simulink model "Model_6DOF_B3"  (R2020b)
settings: Solver=FixedStepAuto  StartTime=0.0  StopTime=120  FixedStep=0.05  RelTol=1e-3
values from neighbouring files (symbols this model uses):
  Ba_0 = [0 0 0 0 0 0]    [ctrl_mode_param.m]
  Bb = 4418825.3321    [load_data.m]
  Bv_0 = [tgt_speed 0 0 0 0 0]    [ctrl_mode_param.m]
  Bx_0 = [0 0 tgt_depth 0 0 0]    [ctrl_mode_param.m]
  Ixx = 5.23e7    (= 52300000)    [load_data.m]
  Ixy = 0    [load_data.m]
  Ixz = 0    [load_data.m]
  Iyy = 1.375e9    (= 1375000000)    [load_data.m]
  Iyz = 0    [load_data.m]
  Izz = 1.367e9    (= 1367000000)    [load_data.m]
  Mb = 4418825.3321    [load_data.m]
  Xb = 0    [load_data.m]
  Xg = 0    [load_data.m]
  Yb = 0    [load_data.m]
  Yg = 0    [load_data.m]
  Zb = 0.4406    [load_data.m]
  Zg = 0    [load_data.m]
undefined symbols (not defined in the file or in its folder): dA_BP1, dA_BP2, dA_Hull, dA_PH, dA_Sail, dA_SProot, dA_X1a, dA_X1b, dA_X2a, dA_X2b, dA_X3a, dA_X3b, dA_X4a, dA_X4b, its, n_BP1, n_BP2, n_Hull, n_PH, n_Sail, n_SProot, n_X1a, n_X1b, n_X2a, n_X2b, n_X3a, n_X3b, n_X4a, n_X4b, nt_BP1, nt_BP2, nt_Hull, nt_PH, nt_Sail, nt_SProot, nt_X1a, nt_X1b, nt_X2a, nt_X2b, nt_X3a, nt_X3b, nt_X4a, nt_X4b, Usp, vt1_BP1, vt1_BP2, vt1_Hull, vt1_PH, vt1_Sail, vt1_SProot, vt1_X1a, vt1_X1b, vt1_X2a, vt1_X2b, vt1_X3a, vt1_X3b, vt1_X4a, vt1_X4b, vt2_BP1, vt2_BP2 ... (+27)
libraries: simulink x5
(part 1 of 15)
settings Model: OrderedModelArguments=off  Creator=yagkim  LastModifiedBy=cooki
settings DebuggingCC: UnderSpecifiedDimensionMsg=warning
settings SFSimCC: CustomCodeUndefinedFunction=UseInterfaceOnly

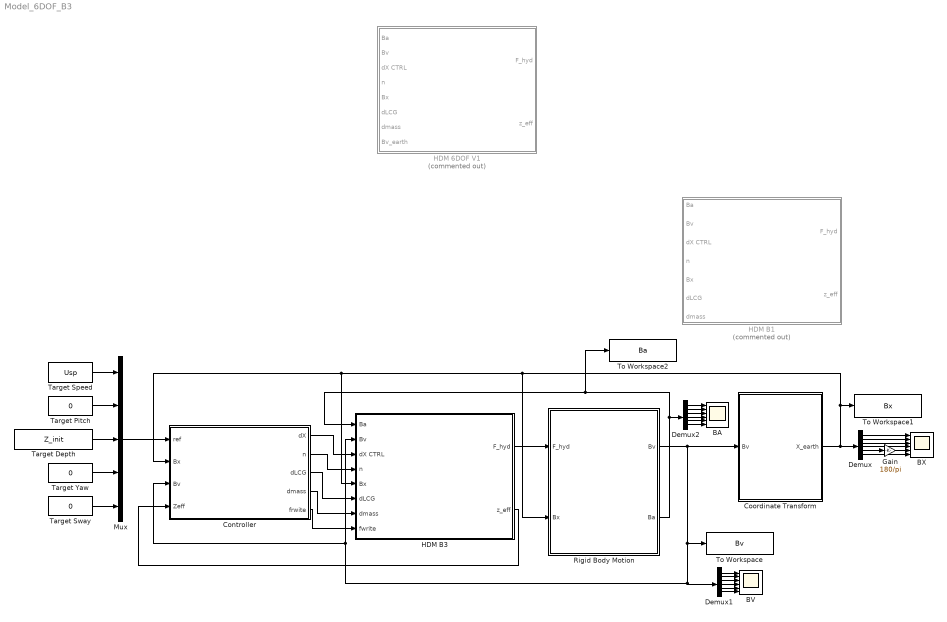
== system Model_6DOF_B3 ==
  BA : Scope  NumInputPorts=6
  BV : Scope  NumInputPorts=6
  BX : Scope  NumInputPorts=6
  Controller : Subsystem
  Coordinate Transform : Subsystem
  Demux : Demux  Outputs=6
  Demux1 : Demux  Outputs=6
  Demux2 : Demux  Outputs=6
  Gain : Gain  Gain=180/pi
  HDM 6DOF V1 : Subsystem  Commented=on  InitFcn='main'
  HDM B1 : Subsystem  Commented=on  InitFcn='main'
  HDM B3 : Subsystem  InitFcn='main'
  Mux : Mux  Inputs=5
  Rigid Body Motion : Subsystem
  Target Depth : Constant  Value=Z_init
  Target Pitch : Constant  Value=0
  Target Speed : Constant  Value=Usp
  Target Sway : Constant  Value=0
  Target Yaw : Constant  Value=0
  To Workspace : ToWorkspace  VariableName=Bv  SaveFormat=Timeseries  SampleTime=-1
  To Workspace1 : ToWorkspace  VariableName=Bx  SaveFormat=Timeseries  SampleTime=-1
  To Workspace2 : ToWorkspace  VariableName=Ba  SaveFormat=Timeseries  SampleTime=-1
  wires:
  Demux/1 -> BX/1
  Demux/2 -> BX/2
  Demux/3 -> BX/3
  Demux/4 -> BX/4
  Demux/6 -> BX/6
  Demux1/6 -> BV/6
  Demux1/5 -> BV/5
  Demux1/4 -> BV/4
  Demux1/3 -> BV/3
  Demux1/2 -> BV/2
  Demux1/1 -> BV/1
  Mux/1 -> Controller/1(ref)
  Target Speed/1 -> Mux/1
  Target Depth/1 -> Mux/3
  Gain/1 -> BX/5
  Demux/5 -> Gain/1
  Controller/2(n) -> HDM B3/4(n)
  Demux2/4 -> BA/4
  Demux2/1 -> BA/1
  Demux2/3 -> BA/3
  Demux2/6 -> BA/6
  Demux2/5 -> BA/5
  Demux2/2 -> BA/2
  Rigid Body Motion/2(Ba) -> To Workspace2/1, HDM B3/1(Ba), Demux2/1
  Rigid Body Motion/1(Bv) -> Coordinate Transform/1(Bv), Demux1/1, HDM B3/2(Bv), Controller/3(Bv), To Workspace/1
  HDM B3/1(F_hyd) -> Rigid Body Motion/1(F_hyd)
  Target Pitch/1 -> Mux/2
  Target Yaw/1 -> Mux/4
  Target Sway/1 -> Mux/5
  Coordinate Transform/1(X_earth) -> Demux/1, Rigid Body Motion/2(Bx), Controller/2(Bx), HDM B3/5(Bx), To Workspace1/1
  Controller/1(dX) -> HDM B3/3(dX CTRL)
  Controller/3(dLCG) -> HDM B3/6(dLCG)
  Controller/4(dmass) -> HDM B3/7(dmass)
  HDM B3/2(z_eff) -> Controller/4(Zeff)
  Controller/5(frwite) -> HDM B3/8(fwrite)

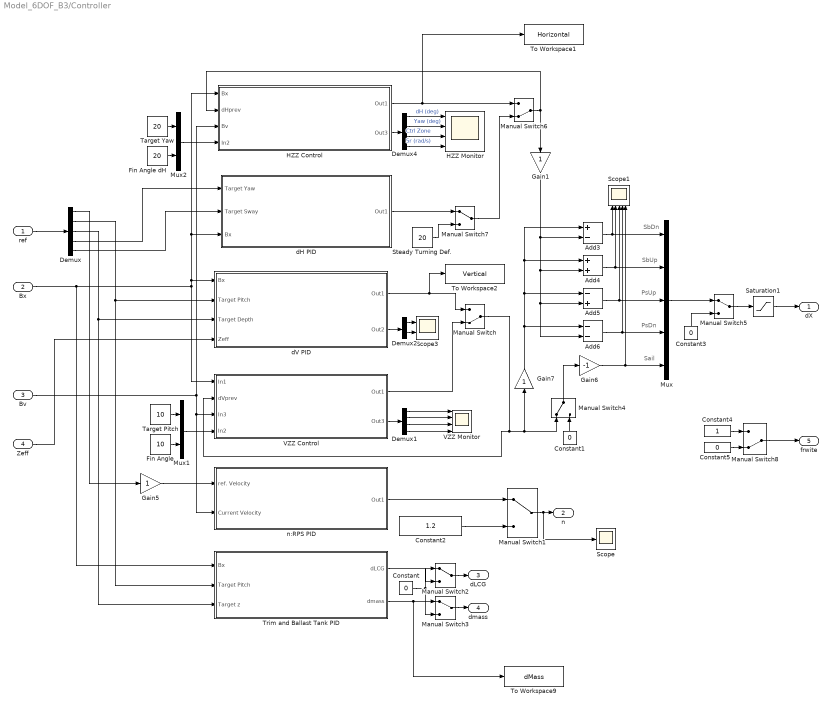
== system Model_6DOF_B3/Controller ==
  note: SbDn
  note: SbUp
  note: PsUp
  note: PsDn
  note: Sail
  ref : Inport
  Bx : Inport  Port=2
  Bv : Inport  Port=3
  Zeff : Inport  Port=4
  Add3 : Sum  Inputs=+-
  Add4 : Sum
  Add5 : Sum  Inputs=-+
  Add6 : Sum  Inputs=--
  Constant{,1,3,5} (4 alike) : Constant  Value=0
  Constant2 : Constant  Value=1.2
  Constant4 : Constant
  Demux : Demux  Outputs=5
  Demux1 : Demux
  Demux2 : Demux  Outputs=2
  Demux4 : Demux
  Fin Angle : Constant  Value=10
  Fin Angle dH : Constant  Value=20
  Gain1 : Gain
  Gain5 : Gain
  Gain6 : Gain  Gain=-1
  Gain7 : Gain
  HZZ Control : Subsystem
  HZZ Monitor : Scope  NumInputPorts=4
  Manual Switch : ManualSwitch  CurrentSetting=0
  Manual Switch{1..5,7} (6 alike) : ManualSwitch
  Manual Switch6 : ManualSwitch  CurrentSetting=0
  Manual Switch8 : ManualSwitch  CurrentSetting=0
  Mux : Mux  Inputs=5
  Mux1 : Mux  Inputs=2
  Mux2 : Mux  Inputs=2
  Saturation1 : Saturate  UpperLimit=30  LowerLimit=-30
  Scope : Scope
  Scope1 : Scope  NumInputPorts=5
  Scope3 : Scope  NumInputPorts=2
  Steady Turning Def. : Constant  Value=20
  Target Pitch : Constant  Value=10
  Target Yaw : Constant  Value=20
  To Workspace1 : ToWorkspace  VariableName=Horizontal  SaveFormat=Timeseries  SampleTime=-1
  To Workspace2 : ToWorkspace  VariableName=Vertical  SaveFormat=Timeseries  SampleTime=-1
  To Workspace9 : ToWorkspace  VariableName=dMass  SaveFormat=Timeseries  SampleTime=-1
  Trim and Ballast Tank PID : Subsystem
  VZZ Control : Subsystem
  VZZ Monitor : Scope  NumInputPorts=4
  dH PID : Subsystem
  dV PID : Subsystem
  n:RPS PID : Subsystem
  dX : Outport  VectorParamsAs1DForOutWhenUnconnected=off
  n : Outport  Port=2  VectorParamsAs1DForOutWhenUnconnected=off
  dLCG : Outport  Port=3  VectorParamsAs1DForOutWhenUnconnected=off
  dmass : Outport  Port=4  VectorParamsAs1DForOutWhenUnconnected=off
  frwite : Outport  Port=5  VectorParamsAs1DForOutWhenUnconnected=off
  wires:
  Add3/1 -> Mux/1, Scope1/1
  Add4/1 -> Mux/2, Scope1/2
  Add5/1 -> Mux/3, Scope1/3
  Add6/1 -> Mux/4, Scope1/4
  Manual Switch6/1 -> HZZ Control/2(dHprev), Gain1/1
  Gain6/1 -> Mux/5, Scope1/5
  Gain7/1 -> Add3/1, Add4/1, Add5/1, Add6/1
  Demux/1 -> Gain5/1
  Bv/1 -> HZZ Control/3(Bv), n:RPS PID/2(Current Velocity), VZZ Control/3(In3)
  Gain5/1 -> n:RPS PID/1(ref. Velocity)
  Constant2/1 -> Manual Switch1/2
  n:RPS PID/1(Out1) -> Manual Switch1/1
  Manual Switch/1 -> VZZ Control/2(dVprev), Manual Switch4/1, Gain7/1
  ref/1 -> Demux/1
  dV PID/1(Out1) -> Manual Switch/1, To Workspace2/1
  Demux/4 -> dH PID/1(Target Yaw)
  Demux/5 -> dH PID/2(Target Sway)
  dH PID/1(Out1) -> Manual Switch7/1
  VZZ Control/1(Out1) -> Manual Switch/2
  Demux1/1 -> VZZ Monitor/1
  Demux1/2 -> VZZ Monitor/2
  Demux1/3 -> VZZ Monitor/3
  Demux1/4 -> VZZ Monitor/4
  VZZ Control/2(Out3) -> Demux1/1
  Mux1/1 -> VZZ Control/4(In2)
  Target Pitch/1 -> Mux1/1
  Fin Angle/1 -> Mux1/2
  Demux/2 -> Trim and Ballast Tank PID/2(Target Pitch), dV PID/2(Target Pitch)
  Bx/1 -> Trim and Ballast Tank PID/1(Bx), HZZ Control/1(Bx), dH PID/3(Bx), dV PID/1(Bx), VZZ Control/1(In1)
  Demux/3 -> Trim and Ballast Tank PID/3(Target z), dV PID/3(Target Depth)
  Trim and Ballast Tank PID/1(dLCG) -> Manual Switch2/2
  Trim and Ballast Tank PID/2(dmass) -> To Workspace9/1, Manual Switch3/1
  Mux/1 -> Manual Switch5/1
  Demux2/2 -> Scope3/2
  Demux2/1 -> Scope3/1
  dV PID/2(Out2) -> Demux2/1
  Manual Switch2/1 -> dLCG/1
  Constant/1 -> Manual Switch3/2, Manual Switch2/1
  Manual Switch4/1 -> Gain6/1
  Constant1/1 -> Manual Switch4/2
  Manual Switch5/1 -> Saturation1/1
  Constant3/1 -> Manual Switch5/2
  Fin Angle dH/1 -> Mux2/2
  Mux2/1 -> HZZ Control/4(In2)
  Target Yaw/1 -> Mux2/1
  Demux4/3 -> HZZ Monitor/3  "Ctrl Zone"
  HZZ Control/2(Out3) -> Demux4/1
  Demux4/4 -> HZZ Monitor/4  "5r (rad/s)"
  Demux4/2 -> HZZ Monitor/2  "Yaw (deg)"
  Demux4/1 -> HZZ Monitor/1  "dH (deg)"
  HZZ Control/1(Out1) -> To Workspace1/1, Manual Switch6/1
  Gain1/1 -> Add6/2, Add5/2, Add4/2, Add3/2
  Zeff/1 -> dV PID/4(Zeff)
  Saturation1/1 -> dX/1
  Manual Switch1/1 -> Scope/1, n/1
  Manual Switch3/1 -> dmass/1
  Manual Switch7/1 -> Manual Switch6/2
  Steady Turning Def./1 -> Manual Switch7/2
  Manual Switch8/1 -> frwite/1
  Constant4/1 -> Manual Switch8/1
  Constant5/1 -> Manual Switch8/2

== system Model_6DOF_B3/Coordinate Transform ==
  Bv : Inport
  Demux : Demux  Outputs=6
  Gain2 : Gain
  Gain6 : Gain
  Integrator : Integrator  InitialCondition=Bx_0
  MATLAB Function2 : MATLAB Function  TreatAsAtomicUnit=on
  Mux : Mux  Inputs=6
  X_earth : Outport  VectorParamsAs1DForOutWhenUnconnected=off
  wires:
  Bv/1 -> MATLAB Function2/2(Bv)
  MATLAB Function2/1(out) -> Integrator/1
  Integrator/1 -> MATLAB Function2/1(Bx), Demux/1
  Mux/1 -> X_earth/1
  Demux/1 -> Mux/1
  Demux/2 -> Mux/2
  Demux/3 -> Gain6/1
  Demux/4 -> Mux/4
  Demux/5 -> Gain2/1
  Demux/6 -> Mux/6
  Gain6/1 -> Mux/3
  Gain2/1 -> Mux/5

== system Model_6DOF_B3/HDM 6DOF V1 ==
  Ba : Inport
  Bv : Inport  Port=2
  dX CTRL : Inport  Port=3
  n : Inport  Port=4
  Bx : Inport  Port=5
  dLCG : Inport  Port=6
  dmass : Inport  Port=7
  Bv_earth : Inport  Port=8
  Constant4 : Constant  Value=0
  Effective Veloicity Calclation : Subsystem
  Effective dX Calculation : Subsystem
  K : Subsystem
  M : Subsystem
  M 6d org : Subsystem  Commented=on
  Manual Switch1 : ManualSwitch
  Manual Switch2 : ManualSwitch
  Manual Switch3 : ManualSwitch  CurrentSetting=0
  Manual Switch4 : ManualSwitch  CurrentSetting=0
  Manual Switch5 : ManualSwitch
  Mux2 : Mux  Inputs=6
  N : Subsystem
  Sea State : Constant  Value=0
  To Workspace1 : ToWorkspace  VariableName=dXeff  SaveFormat=Timeseries  SampleTime=-1
  To Workspace2 : ToWorkspace  VariableName=AOA  SaveFormat=Timeseries  SampleTime=-1
  Wave Particle Velocity : Subsystem
  X : Subsystem
  X 6d org : Subsystem  Commented=on
  Y : Subsystem
  Z : Subsystem
  Z 6d org : Subsystem  Commented=on
  alpha : Scope
  dXeff : Scope
  F_hyd : Outport  VectorParamsAs1DForOutWhenUnconnected=off
  z_eff : Outport  Port=2  VectorParamsAs1DForOutWhenUnconnected=off
  wires:
  Constant4/1 -> Manual Switch4/2, Manual Switch3/2, Manual Switch1/1, Manual Switch2/1, Manual Switch5/1
  Mux2/1 -> F_hyd/1
  X/1(X) -> Mux2/1
  Manual Switch3/1 -> Mux2/3
  Manual Switch2/1 -> Mux2/5
  Effective dX Calculation/1(dXeff) -> To Workspace1/1, dXeff/1, X/5(dXeff), M/6(dX), K/6(dX), Z/6(dX), N/6(dX), Y/6(dX)
  Ba/1 -> X/3(Ba), Y/3(Ba), K/3(Ba), Z/3(Ba), M/3(Ba), N/3(Ba)
  M/1(M) -> Manual Switch2/2
  Z/1(Z) -> Manual Switch3/1
  dX CTRL/1 -> X/12(dXraw), Effective dX Calculation/1(dX CTRL)
  Bx/1 -> X/1(Bx), N/1(Bx), K/1(Bx), Y/1(Bx), Z/1(Bx), M/1(Bx), Wave Particle Velocity/1(Bx_earth)
  dLCG/1 -> Wave Particle Velocity/5(dLCG), X/9(dLCG), Z/8(dLCG), N/8(dLCG), M/8(dLCG), K/8(dLCG), Y/8(dLCG)
  dmass/1 -> M/9(dmass), N/9(dmass), K/9(dmass), Z/9(dmass), Y/9(dmass), X/10(dmass)
  Bv/1 -> Z/2(Bv), N/2(Bv), K/2(Bv), Y/2(Bv), Effective Veloicity Calclation/1(Bv), X/2(Bv), M/2(Bv), Wave Particle Velocity/3(Bv_ship)
  Bv_earth/1 -> Wave Particle Velocity/2(Bv_earth)
  Sea State/1 -> Wave Particle Velocity/4(SeaState)
  Wave Particle Velocity/7(z_eff) -> z_eff/1
  N/1(N) -> Manual Switch1/2
  Y/1(Y) -> Manual Switch4/1
  Manual Switch4/1 -> Mux2/2
  Manual Switch1/1 -> Mux2/6
  Manual Switch5/1 -> Mux2/4
  K/1(K) -> Manual Switch5/2
  Wave Particle Velocity/2(Yvm) -> Y/10(Yvm)
  Wave Particle Velocity/4(Kvm) -> K/10(Kvm)
  Wave Particle Velocity/6(Nvm) -> N/10(Nvm)
  Wave Particle Velocity/8(uwsXi) -> Effective Veloicity Calclation/2(uwsXi)
  Wave Particle Velocity/9(uwsCG) -> Effective Veloicity Calclation/3(uwsCG)
  Effective Veloicity Calclation/5(UeX) -> Y/7(UeX), X/6(UeSP), Z/7(UeSP), N/7(UeX), K/7(UeX), M/7(UeSP)
  Effective Veloicity Calclation/3(Umag) -> Y/5(Umag), M/5(Umag), Z/5(Umag), X/4(Umag), K/5(Umag), N/5(Umag)
  Effective Veloicity Calclation/1(Alpha) -> alpha/1, To Workspace2/1, Z/4(Alpha), M/4(Alpha), X/8(Alpha)
  Effective Veloicity Calclation/2(Beta) -> N/4(Beta), K/4(Beta), Y/4(Beta)
  Effective Veloicity Calclation/4(aXi) -> X/11(dXadd), Effective dX Calculation/2(aXi)
  Wave Particle Velocity/1(Xvm) -> X/13(Xvm)
  n/1 -> X/7(n)
  Wave Particle Velocity/3(Zvm) -> Z/10(Zvm)
  Wave Particle Velocity/5(Mvm) -> M/10(Mvm)

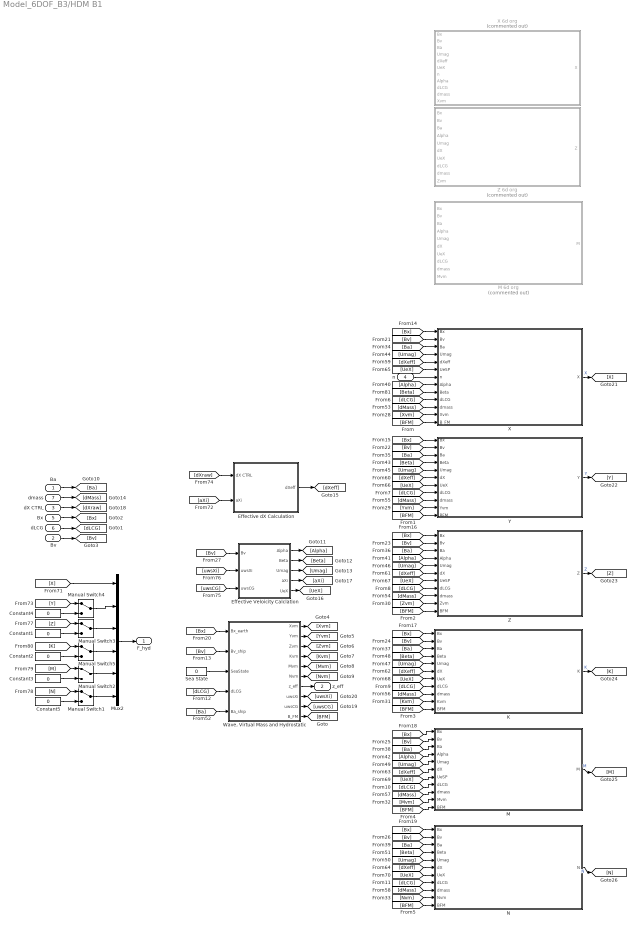
== system Model_6DOF_B3/HDM B1 ==
  Ba : Inport
  Bv : Inport  Port=2
  dX CTRL : Inport  Port=3
  n : Inport  Port=4
  Bx : Inport  Port=5
  dLCG : Inport  Port=6
  dmass : Inport  Port=7
  Constant{1..5} (5 alike) : Constant  Value=0
  Effective Veloicity Calclation : Subsystem
  Effective dX Calculation : Subsystem
  K : Subsystem
  M : Subsystem
  M 6d org : Subsystem  Commented=on
  Manual Switch{1..5} (5 alike) : ManualSwitch
  Mux2 : Mux  Inputs=6
  N : Subsystem
  Sea State : Constant  Value=0
  "Wave, Virtual Mass and Hydrostatic" : Subsystem
  X : Subsystem
  X 6d org : Subsystem  Commented=on
  Y : Subsystem
  Z : Subsystem
  Z 6d org : Subsystem  Commented=on
  F_hyd : Outport  VectorParamsAs1DForOutWhenUnconnected=off
  z_eff : Outport  Port=2  VectorParamsAs1DForOutWhenUnconnected=off
  wires:
  [Beta] -> X/9(Beta)
  [K] -> Manual Switch5/1
  [M] -> Manual Switch2/1
  [N] -> Manual Switch1/1
  [Z] -> Manual Switch3/1
  [Y] -> Manual Switch4/1
  Constant5/1 -> Manual Switch1/2
  Constant3/1 -> Manual Switch2/2
  Constant2/1 -> Manual Switch5/2
  Constant1/1 -> Manual Switch3/2
  Constant4/1 -> Manual Switch4/2
  [X] -> Mux2/1
  N/1(N) -> [N]  "N"
  M/1(M) -> [M]  "M"
  K/1(K) -> [K]  "K"
  Z/1(Z) -> [Z]  "Z"
  Y/1(Y) -> [Y]  "Y"
  X/1(X) -> [X]  "X"
  [uwsXi] -> Effective Veloicity Calclation/2(uwsXi)
  "Wave, Virtual Mass and Hydrostatic"/8(uwsXi) -> [uwsXi]
  [uwsCG] -> Effective Veloicity Calclation/3(uwsCG)
  "Wave, Virtual Mass and Hydrostatic"/9(uwsCG) -> [uwsCG]
  [dXraw] -> Effective dX Calculation/1(dX CTRL)
  dX CTRL/1 -> [dXraw]
  [aXi] -> Effective dX Calculation/2(aXi)
  Effective Veloicity Calclation/4(aXi) -> [aXi]
  [UeX] -> N/7(UeX)
  [UeX] -> M/7(UeSP)
  [UeX] -> K/7(UeX)
  [UeX] -> Z/7(UeSP)
  [UeX] -> Y/7(UeX)
  [UeX] -> X/6(UeSP)
  Effective Veloicity Calclation/5(UeX) -> [UeX]
  [dXeff] -> N/6(dX)
  [dXeff] -> M/6(dX)
  [dXeff] -> K/6(dX)
  [dXeff] -> Z/6(dX)
  [dXeff] -> Y/6(dX)
  [dXeff] -> X/5(dXeff)
  [dMass] -> N/9(dmass)
  [dMass] -> M/9(dmass)
  [dMass] -> K/9(dmass)
  [dMass] -> Y/9(dmass)
  [dMass] -> Z/9(dmass)
  [dMass] -> X/11(dmass)
  [Ba] -> "Wave, Virtual Mass and Hydrostatic"/5(Ba_ship)
  dmass/1 -> [dMass]
  [Beta] -> N/4(Beta)
  [Umag] -> N/5(Umag)
  [Umag] -> M/5(Umag)
  [Beta] -> K/4(Beta)
  [Umag] -> K/5(Umag)
  [Umag] -> Z/5(Umag)
  [Umag] -> Y/5(Umag)
  [Umag] -> X/4(Umag)
  Effective Veloicity Calclation/3(Umag) -> [Umag]
  [Beta] -> Y/4(Beta)
  Effective Veloicity Calclation/2(Beta) -> [Beta]
  [Alpha] -> M/4(Alpha)
  [Alpha] -> Z/4(Alpha)
  [Alpha] -> X/8(Alpha)
  Effective Veloicity Calclation/1(Alpha) -> [Alpha]
  [Ba] -> N/3(Ba)
  [Ba] -> M/3(Ba)
  [Ba] -> K/3(Ba)
  [Ba] -> Z/3(Ba)
  [Ba] -> Y/3(Ba)
  [Ba] -> X/3(Ba)
  [Nvm] -> N/10(Nvm)
  [Mvm] -> M/10(Mvm)
  [Kvm] -> K/10(Kvm)
  [Bv] -> Z/2(Bv)
  [Zvm] -> Z/10(Zvm)
  [Yvm] -> Y/10(Yvm)
  [Xvm] -> X/12(Xvm)
  "Wave, Virtual Mass and Hydrostatic"/6(Nvm) -> [Nvm]
  "Wave, Virtual Mass and Hydrostatic"/5(Mvm) -> [Mvm]
  "Wave, Virtual Mass and Hydrostatic"/4(Kvm) -> [Kvm]
  "Wave, Virtual Mass and Hydrostatic"/3(Zvm) -> [Zvm]
  "Wave, Virtual Mass and Hydrostatic"/2(Yvm) -> [Yvm]
  "Wave, Virtual Mass and Hydrostatic"/1(Xvm) -> [Xvm]
  [Bv] -> Effective Veloicity Calclation/1(Bv)
  [Bv] -> N/2(Bv)
  [Bv] -> M/2(Bv)
  [Bv] -> K/2(Bv)
  [Bv] -> Y/2(Bv)
  [Bv] -> X/2(Bv)
  [Bv] -> "Wave, Virtual Mass and Hydrostatic"/2(Bv_ship)
  [Bx] -> "Wave, Virtual Mass and Hydrostatic"/1(Bx_earth)
  [Bx] -> N/1(Bx)
  [Bx] -> M/1(Bx)
  [Bx] -> K/1(Bx)
  [Bx] -> Z/1(Bx)
  [Bx] -> Y/1(Bx)
  [Bx] -> X/1(Bx)
  [dLCG] -> "Wave, Virtual Mass and Hydrostatic"/4(dLCG)
  [dLCG] -> N/8(dLCG)
  [dLCG] -> M/8(dLCG)
  [dLCG] -> K/8(dLCG)
  [dLCG] -> Z/8(dLCG)
  [dLCG] -> Y/8(dLCG)
  [dLCG] -> X/10(dLCG)
  [BFM] -> N/11(BFM)
  [BFM] -> M/11(BFM)
  [BFM] -> K/11(BFM)
  [BFM] -> Z/11(BFM)
  [BFM] -> Y/11(BFM)
  [BFM] -> X/13(B_FM)
  "Wave, Virtual Mass and Hydrostatic"/10(B_FM) -> [BFM]
  n/1 -> X/7(n)
  Manual Switch5/1 -> Mux2/4
  Manual Switch1/1 -> Mux2/6
  Manual Switch4/1 -> Mux2/2
  "Wave, Virtual Mass and Hydrostatic"/7(z_eff) -> z_eff/1
  Sea State/1 -> "Wave, Virtual Mass and Hydrostatic"/3(SeaState)
  Bv/1 -> [Bv]
  dLCG/1 -> [dLCG]
  Bx/1 -> [Bx]
  Ba/1 -> [Ba]
  Effective dX Calculation/1(dXeff) -> [dXeff]
  Manual Switch2/1 -> Mux2/5
  Manual Switch3/1 -> Mux2/3
  Mux2/1 -> F_hyd/1

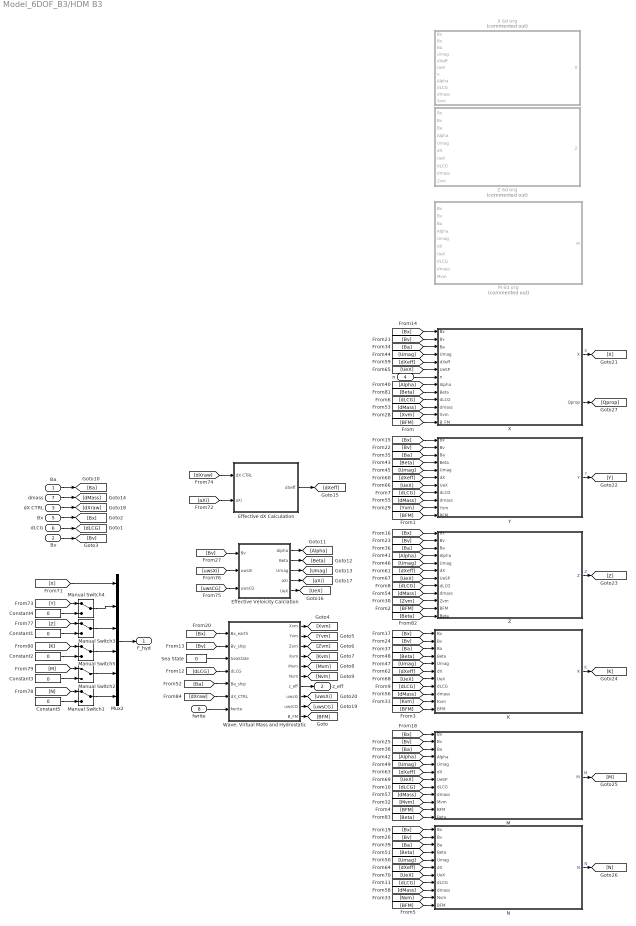
== system Model_6DOF_B3/HDM B3 ==
  Ba : Inport
  Bv : Inport  Port=2
  dX CTRL : Inport  Port=3
  n : Inport  Port=4
  Bx : Inport  Port=5
  dLCG : Inport  Port=6
  dmass : Inport  Port=7
  fwrite : Inport  Port=8
  Constant{1..5} (5 alike) : Constant  Value=0
  Effective Veloicity Calclation : Subsystem
  Effective dX Calculation : Subsystem
  K : Subsystem
  M : Subsystem
  M 6d org : Subsystem  Commented=on
  Manual Switch{1..5} (5 alike) : ManualSwitch
  Mux2 : Mux  Inputs=6
  N : Subsystem
  Sea State : Constant  Value=0
  "Wave, Virtual Mass and Hydrostatic" : Subsystem
  X : Subsystem
  X 6d org : Subsystem  Commented=on
  Y : Subsystem
  Z : Subsystem
  Z 6d org : Subsystem  Commented=on
  F_hyd : Outport  VectorParamsAs1DForOutWhenUnconnected=off
  z_eff : Outport  Port=2  VectorParamsAs1DForOutWhenUnconnected=off
  wires:
  Mux2/1 -> F_hyd/1
  Manual Switch3/1 -> Mux2/3
  Manual Switch2/1 -> Mux2/5
  Effective dX Calculation/1(dXeff) -> [dXeff]
  Ba/1 -> [Ba]
  Bx/1 -> [Bx]
  dLCG/1 -> [dLCG]
  Bv/1 -> [Bv]
  Sea State/1 -> "Wave, Virtual Mass and Hydrostatic"/3(SeaState)
  "Wave, Virtual Mass and Hydrostatic"/7(z_eff) -> z_eff/1
  Manual Switch4/1 -> Mux2/2
  Manual Switch1/1 -> Mux2/6
  Manual Switch5/1 -> Mux2/4
  n/1 -> X/7(n)
  "Wave, Virtual Mass and Hydrostatic"/10(B_FM) -> [BFM]
  [BFM] -> X/13(B_FM)
  [BFM] -> Y/11(BFM)
  [BFM] -> Z/11(BFM)
  [BFM] -> K/11(BFM)
  [BFM] -> M/11(BFM)
  [BFM] -> N/11(BFM)
  [dLCG] -> X/10(dLCG)
  [dLCG] -> Y/8(dLCG)
  [dLCG] -> Z/8(dLCG)
  [dLCG] -> K/8(dLCG)
  [dLCG] -> M/8(dLCG)
  [dLCG] -> N/8(dLCG)
  [dLCG] -> "Wave, Virtual Mass and Hydrostatic"/4(dLCG)
  [Bx] -> X/1(Bx)
  [Bx] -> Y/1(Bx)
  [Bx] -> Z/1(Bx)
  [Bx] -> K/1(Bx)
  [Bx] -> M/1(Bx)
  [Bx] -> N/1(Bx)
  [Bx] -> "Wave, Virtual Mass and Hydrostatic"/1(Bx_earth)
  [Bv] -> "Wave, Virtual Mass and Hydrostatic"/2(Bv_ship)
  [Bv] -> X/2(Bv)
  [Bv] -> Y/2(Bv)
  [Bv] -> K/2(Bv)
  [Bv] -> M/2(Bv)
  [Bv] -> N/2(Bv)
  [Bv] -> Effective Veloicity Calclation/1(Bv)
  "Wave, Virtual Mass and Hydrostatic"/1(Xvm) -> [Xvm]
  "Wave, Virtual Mass and Hydrostatic"/2(Yvm) -> [Yvm]
  "Wave, Virtual Mass and Hydrostatic"/3(Zvm) -> [Zvm]
  "Wave, Virtual Mass and Hydrostatic"/4(Kvm) -> [Kvm]
  "Wave, Virtual Mass and Hydrostatic"/5(Mvm) -> [Mvm]
  "Wave, Virtual Mass and Hydrostatic"/6(Nvm) -> [Nvm]
  [Xvm] -> X/12(Xvm)
  [Yvm] -> Y/10(Yvm)
  [Zvm] -> Z/10(Zvm)
  [Bv] -> Z/2(Bv)
  [Kvm] -> K/10(Kvm)
  [Mvm] -> M/10(Mvm)
  [Nvm] -> N/10(Nvm)
  [Ba] -> X/3(Ba)
  [Ba] -> Y/3(Ba)
  [Ba] -> Z/3(Ba)
  [Ba] -> K/3(Ba)
  [Ba] -> M/3(Ba)
  [Ba] -> N/3(Ba)
  Effective Veloicity Calclation/1(Alpha) -> [Alpha]
  [Alpha] -> X/8(Alpha)
  [Alpha] -> Z/4(Alpha)
  [Alpha] -> M/4(Alpha)
  Effective Veloicity Calclation/2(Beta) -> [Beta]
  [Beta] -> Y/4(Beta)
  Effective Veloicity Calclation/3(Umag) -> [Umag]
  [Umag] -> X/4(Umag)
  [Umag] -> Y/5(Umag)
  [Umag] -> Z/5(Umag)
  [Umag] -> K/5(Umag)
  [Beta] -> K/4(Beta)
  [Umag] -> M/5(Umag)
  [Umag] -> N/5(Umag)
  [Beta] -> N/4(Beta)
  dmass/1 -> [dMass]
  [Ba] -> "Wave, Virtual Mass and Hydrostatic"/5(Ba_ship)
  [dMass] -> X/11(dmass)
  [dMass] -> Z/9(dmass)
  [dMass] -> Y/9(dmass)
  [dMass] -> K/9(dmass)
  [dMass] -> M/9(dmass)
  [dMass] -> N/9(dmass)
  [dXeff] -> X/5(dXeff)
  [dXeff] -> Y/6(dX)
  [dXeff] -> Z/6(dX)
  [dXeff] -> K/6(dX)
  [dXeff] -> M/6(dX)
  [dXeff] -> N/6(dX)
  Effective Veloicity Calclation/5(UeX) -> [UeX]
  [UeX] -> X/6(UeSP)
  [UeX] -> Y/7(UeX)
  [UeX] -> Z/7(UeSP)
  [UeX] -> K/7(UeX)
  [UeX] -> M/7(UeSP)
  [UeX] -> N/7(UeX)
  Effective Veloicity Calclation/4(aXi) -> [aXi]
  [aXi] -> Effective dX Calculation/2(aXi)
  dX CTRL/1 -> [dXraw]
  [dXraw] -> Effective dX Calculation/1(dX CTRL)
  "Wave, Virtual Mass and Hydrostatic"/9(uwsCG) -> [uwsCG]
  [uwsCG] -> Effective Veloicity Calclation/3(uwsCG)
  "Wave, Virtual Mass and Hydrostatic"/8(uwsXi) -> [uwsXi]
  [uwsXi] -> Effective Veloicity Calclation/2(uwsXi)
  X/1(X) -> [X]  "X"
  Y/1(Y) -> [Y]  "Y"
  Z/1(Z) -> [Z]  "Z"
  K/1(K) -> [K]  "K"
  M/1(M) -> [M]  "M"
  N/1(N) -> [N]  "N"
  [X] -> Mux2/1
  Constant4/1 -> Manual Switch4/2
  Constant1/1 -> Manual Switch3/2
  Constant2/1 -> Manual Switch5/2
  Constant3/1 -> Manual Switch2/2
  Constant5/1 -> Manual Switch1/2
  [Y] -> Manual Switch4/1
  [Z] -> Manual Switch3/1
  [N] -> Manual Switch1/1
  [M] -> Manual Switch2/1
  [K] -> Manual Switch5/1
  [Beta] -> X/9(Beta)
  [Beta] -> Z/12(Beta)
  [Beta] -> M/12(Beta)
  [dXraw] -> "Wave, Virtual Mass and Hydrostatic"/6(dX_CTRL)
  fwrite/1 -> "Wave, Virtual Mass and Hydrostatic"/7(fwrite)
  X/2(Qprop) -> [Qprop]

== system Model_6DOF_B3/Rigid Body Motion ==
  F_hyd : Inport
  Bx : Inport  Port=2
  Demux : Demux  Outputs=6
  Demux1 : Demux  Outputs=6
  Demux2 : Demux  Outputs=5
  Gain2 : Gain
  Integrator : Integrator  InitialCondition=Bv_0
  MATLAB Function2 : MATLAB Function  TreatAsAtomicUnit=on
  Memory1 : Memory  InitialCondition=Ba_0
  Mux1 : Mux  Inputs=6
  Mux2 : Mux  Inputs=5
  Bv : Outport  VectorParamsAs1DForOutWhenUnconnected=off
  Ba : Outport  Port=2  VectorParamsAs1DForOutWhenUnconnected=off
  wires:
  Bx/1 -> MATLAB Function2/7(bx)
  MATLAB Function2/1(out) -> Integrator/1, Memory1/1
  Integrator/1 -> MATLAB Function2/8(bv), Demux1/1
  Memory1/1 -> Ba/1
  Demux/1 -> MATLAB Function2/1(X)
  Demux/2 -> MATLAB Function2/2(Y)
  Demux/3 -> MATLAB Function2/3(Z)
  Demux/4 -> MATLAB Function2/4(K)
  Demux/5 -> MATLAB Function2/5(M)
  Demux/6 -> MATLAB Function2/6(N)
  F_hyd/1 -> Demux/1
  Demux2/3 -> Mux1/4
  Demux1/3 -> Mux2/2
  Mux2/1 -> Gain2/1
  Demux2/5 -> Mux1/6
  Demux2/2 -> Mux1/3
  Demux2/4 -> Mux1/5
  Demux1/1 -> Mux1/1
  Demux2/1 -> Mux1/2
  Demux1/5 -> Mux2/4
  Demux1/6 -> Mux2/5
  Demux1/4 -> Mux2/3
  Demux1/2 -> Mux2/1
  Gain2/1 -> Demux2/1
  Mux1/1 -> Bv/1

== system Model_6DOF_B3/Controller/HZZ Control ==
  Bx : Inport
  dHprev : Inport  Port=2
  Bv : Inport  Port=3
  In2 : Inport  Port=4
  Clock : Clock
  Demux : Demux  Outputs=2
  Gain1 : Gain  Gain=-1
  Gain10 : Gain  Gain=180/pi
  Gain11 : Gain  Gain=5
  Gain2 : Gain
  Gain3 : Gain
  Gain4 : Gain
  Gain8 : Gain  Gain=180/pi
  Integrator2 : Integrator
  MATLAB Function : MATLAB Function  TreatAsAtomicUnit=on
  Max Fin Rate : Constant  Value=7.11
  Mux2 : Mux
  Saturation4 : Saturate  UpperLimit=20  LowerLimit=-20
  Selector2 : Selector  InputPortWidth=6  IndexOptions=Index vector (dialog)  Indices=6  OutputSizes=1
  Selector3 : Selector  InputPortWidth=6  IndexOptions=Index vector (dialog)  Indices=6  OutputSizes=1
  Out1 : Outport
  Out3 : Outport  Port=2
  wires:
  Gain11/1 -> Mux2/4
  Selector3/1 -> Gain10/1
  MATLAB Function/1(dVrate) -> Integrator2/1
  MATLAB Function/2(zone) -> Mux2/3
  Gain10/1 -> Gain11/1
  Max Fin Rate/1 -> MATLAB Function/1(rate)
  dHprev/1 -> Gain2/1
  Selector2/1 -> Gain8/1
  Clock/1 -> MATLAB Function/2(trigger)
  Gain8/1 -> Gain3/1
  Bx/1 -> Selector2/1
  Integrator2/1 -> Saturation4/1
  Saturation4/1 -> MATLAB Function/4(dVprev), Gain1/1
  Bv/1 -> Selector3/1
  Mux2/1 -> Out3/1
  In2/1 -> Gain4/1
  Demux/1 -> MATLAB Function/5(dVmax)
  Demux/2 -> MATLAB Function/6(dXmax)
  Gain1/1 -> Out1/1
  Gain2/1 -> Mux2/1
  Gain4/1 -> Demux/1
  Gain3/1 -> MATLAB Function/3(X5), Mux2/2

== system Model_6DOF_B3/Controller/Trim and Ballast Tank PID ==
  Bx : Inport
  Target Pitch : Inport  Port=2
  Target z : Inport  Port=3
  " LCG Change Saturation" : Saturate
  Add : Sum  Inputs=+++
  Add1 : Sum  Inputs=+++
  Add2 : Sum  Inputs=+++
  Add3 : Sum
  Add7 : Sum  Inputs=-+
  Add9 : Sum  Inputs=-+
  Constant2 : Constant  Value=100
  Constant3 : Constant  Value=-100
  D-Depth : Gain  Gain=0
  D-LCG : Gain  Gain=0
  D-mass : Gain  Gain=0
  Derivative : Derivative
  Derivative1 : Derivative
  Derivative2 : Derivative
  Gain36 : Gain  Gain=180/pi
  I-Depth : Gain  Gain=0.00002
  I-LCG : Gain  Gain=0.00002
  I-mass : Gain  Gain=100
  Integrator : Integrator
  Integrator1 : Integrator
  Integrator3 : Integrator
  Lower Rate limit : Constant  Value=-5.83e-4
  Max Mass Change : Saturate  UpperLimit=20000  LowerLimit=-20000
  P-Depth : Gain  Gain=0.00035
  P-LCG : Gain  Gain=0.00035
  P-mass : Gain  Gain=1000
  PID LCG : Selector  InputPortWidth=6  IndexOptions=Index vector (dialog)  Indices=5  OutputSizes=1
  PID mass : Selector  InputPortWidth=6  IndexOptions=Index vector (dialog)  Indices=3  OutputSizes=1
  Rate Limiter Dynamic : simulink/Discontinuities/Rate Limiter Dynamic
  Rate Limiter Dynamic1 : simulink/Discontinuities/Rate Limiter Dynamic
  Upper Rate limit : Constant  Value=5.83e-4
  dLCG : Outport
  dmass : Outport  Port=2
  wires:
  D-mass/1 -> Add/3
  Bx/1 -> PID LCG/1, PID mass/1
  I-mass/1 -> Add/2
  Gain36/1 -> Add9/2  "Pitch (deg)"
  P-LCG/1 -> Add1/1
  D-LCG/1 -> Add1/3
  PID LCG/1 -> Gain36/1
  Rate Limiter Dynamic/1 -> " LCG Change Saturation"/1  "dLCG (m)"
  Integrator/1 -> I-mass/1
  Target z/1 -> Add7/1
  Derivative/1 -> D-mass/1
  PID mass/1 -> Add7/2
  Derivative1/1 -> D-LCG/1
  Integrator3/1 -> I-LCG/1
  I-LCG/1 -> Add1/2
  P-mass/1 -> Add/1
  Target Pitch/1 -> Add9/1
  Upper Rate limit/1 -> Rate Limiter Dynamic/1
  Lower Rate limit/1 -> Rate Limiter Dynamic/3
  Max Mass Change/1 -> dmass/1  "dmass (kg)"
  Add/1 -> Rate Limiter Dynamic1/2
  Rate Limiter Dynamic1/1 -> Max Mass Change/1  "dmass (kg)"
  Constant2/1 -> Rate Limiter Dynamic1/1
  Constant3/1 -> Rate Limiter Dynamic1/3
  " LCG Change Saturation"/1 -> dLCG/1  "dLCG (m)"
  I-Depth/1 -> Add2/2
  Integrator1/1 -> I-Depth/1
  Derivative2/1 -> D-Depth/1
  D-Depth/1 -> Add2/3
  P-Depth/1 -> Add2/1
  Add3/1 -> Rate Limiter Dynamic/2
  Add1/1 -> Add3/1
  Add2/1 -> Add3/2
  Add7/1 -> Derivative/1, Integrator/1, P-Depth/1, Integrator1/1, Derivative2/1, P-mass/1  "e_z (m)"
  Add9/1 -> Derivative1/1, Integrator3/1, P-LCG/1  "e_pitch (deg)"

== system Model_6DOF_B3/Controller/VZZ Control ==
  In1 : Inport
  dVprev : Inport  Port=2
  In3 : Inport  Port=3
  In2 : Inport  Port=4
  Clock : Clock
  Demux : Demux  Outputs=2
  Gain1 : Gain  Gain=-1
  Gain10 : Gain  Gain=180/pi
  Gain11 : Gain  Gain=5
  Gain8 : Gain  Gain=180/pi
  Integrator2 : Integrator
  MATLAB Function : MATLAB Function  TreatAsAtomicUnit=on
  Max Fin Rate : Constant  Value=7.11
  Mux2 : Mux
  Saturation4 : Saturate  UpperLimit=20  LowerLimit=-20
  Selector2 : Selector  InputPortWidth=6  IndexOptions=Index vector (dialog)  Indices=5  OutputSizes=1
  Selector3 : Selector  InputPortWidth=6  IndexOptions=Index vector (dialog)  Indices=5  OutputSizes=1
  Out1 : Outport
  Out3 : Outport  Port=2
  wires:
  Gain11/1 -> Mux2/4
  Selector3/1 -> Gain10/1
  MATLAB Function/1(dVrate) -> Integrator2/1
  MATLAB Function/2(zone) -> Mux2/3
  Gain10/1 -> Gain11/1
  Max Fin Rate/1 -> MATLAB Function/1(rate)
  dVprev/1 -> Mux2/1
  Selector2/1 -> Gain8/1
  Clock/1 -> MATLAB Function/2(trigger)
  Gain8/1 -> MATLAB Function/3(X5), Mux2/2
  In1/1 -> Selector2/1
  Integrator2/1 -> Saturation4/1
  Saturation4/1 -> MATLAB Function/4(dVprev), Gain1/1
  In3/1 -> Selector3/1
  Mux2/1 -> Out3/1
  In2/1 -> Demux/1
  Demux/1 -> MATLAB Function/5(dVmax)
  Demux/2 -> MATLAB Function/6(dXmax)
  Gain1/1 -> Out1/1

== system Model_6DOF_B3/Controller/dH PID ==
  Target Yaw : Inport
  Target Sway : Inport  Port=2
  Bx : Inport  Port=3
  Add1 : Sum  Inputs=+++
  Add10 : Sum
  Add2 : Sum  Inputs=+++
  Add7 : Sum  Inputs=-+
  Add9 : Sum  Inputs=-+
  Constant : Constant  Value=7.11
  Constant1 : Constant  Value=-7.11
  D-Sway : Gain  Gain=0
  D-Yaw : Gain  Gain=12.199
  Derivative : Derivative
  Derivative1 : Derivative
  Gain36 : Gain  Gain=180/pi
  I-Sway : Gain  Gain=0
  I-Yaw : Gain  Gain=0
  Integrator : Integrator
  Integrator3 : Integrator
  Max Deflection : Saturate  UpperLimit=30  LowerLimit=-30
  P-Sway1 : Gain  Gain=-1.452
  P-Yaw : Gain  Gain=3
  PID Sway : Selector  InputPortWidth=6  IndexOptions=Index vector (dialog)  Indices=2  OutputSizes=1
  PID Yaw : Selector  InputPortWidth=6  IndexOptions=Index vector (dialog)  Indices=6  OutputSizes=1
  Rate Limiter Dynamic : simulink/Discontinuities/Rate Limiter Dynamic
  Out1 : Outport
  wires:
  Integrator3/1 -> I-Yaw/1
  Add9/1 -> P-Yaw/1, Derivative1/1, Integrator3/1
  Add2/1 -> Add10/2
  I-Yaw/1 -> Add1/2
  Add7/1 -> P-Sway1/1, Derivative/1, Integrator/1
  Target Sway/1 -> Add7/1
  Derivative/1 -> D-Sway/1
  PID Sway/1 -> Add7/2
  P-Yaw/1 -> Add1/1
  Bx/1 -> PID Yaw/1, PID Sway/1
  I-Sway/1 -> Add2/2
  Rate Limiter Dynamic/1 -> Max Deflection/1
  D-Yaw/1 -> Add1/3
  PID Yaw/1 -> Gain36/1
  Add1/1 -> Add10/1
  Integrator/1 -> I-Sway/1
  Gain36/1 -> Add9/2
  Max Deflection/1 -> Out1/1
  P-Sway1/1 -> Add2/1
  D-Sway/1 -> Add2/3
  Derivative1/1 -> D-Yaw/1
  Add10/1 -> Rate Limiter Dynamic/2
  Target Yaw/1 -> Add9/1
  Constant1/1 -> Rate Limiter Dynamic/3
  Constant/1 -> Rate Limiter Dynamic/1

== system Model_6DOF_B3/Controller/dV PID ==
  Bx : Inport
  Target Pitch : Inport  Port=2
  Target Depth : Inport  Port=3
  Zeff : Inport  Port=4
  Add : Sum  Inputs=+++
  Add1 : Sum  Inputs=+++
  Add10 : Sum
  Add7 : Sum  Inputs=-+
  Add9 : Sum  Inputs=-+
  Constant : Constant  Value=7.11
  Constant1 : Constant  Value=-7.11
  D-Depth : Gain  Gain=3
  D-Pitch : Gain  Gain=3
  Derivative : Derivative
  Derivative3 : Derivative
  Gain36 : Gain  Gain=180/pi
  I-Depth : Gain  Gain=0.1044
  I-Pitch : Gain  Gain=0.1466
  I-Pitch{1..6} (6 alike) : Gain
  Integrator : Integrator
  Integrator3 : Integrator
  Max Deflection : Saturate  UpperLimit=30  LowerLimit=-30
  Mux : Mux  Inputs=2
  P-Depth : Gain  Gain=3
  P-Pitch : Gain  Gain=3
  PID Pitch : Selector  InputPortWidth=6  IndexOptions=Index vector (dialog)  Indices=5  OutputSizes=1
  Rate Limiter Dynamic : simulink/Discontinuities/Rate Limiter Dynamic
  Out1 : Outport
  Out2 : Outport  Port=2
  wires:
  Add/1 -> Mux/2, Add10/2  "dV Depth (deg)"
  Add7/1 -> Derivative3/1, Integrator/1, P-Depth/1  "Erorr in z (m)"
  Zeff/1 -> Add7/2  "z (m)"
  Integrator/1 -> I-Depth/1
  P-Depth/1 -> I-Pitch4/1
  Gain36/1 -> Add9/2  "Pitch (deg)"
  Add9/1 -> Derivative/1, Integrator3/1, P-Pitch/1  "Error in Pitch (deg)"
  P-Pitch/1 -> I-Pitch3/1
  Bx/1 -> PID Pitch/1
  Derivative3/1 -> D-Depth/1
  Add1/1 -> Add10/1, Mux/1  "dV Pitch (deg)"
  D-Depth/1 -> I-Pitch6/1
  Derivative/1 -> D-Pitch/1
  Integrator3/1 -> I-Pitch/1
  PID Pitch/1 -> Gain36/1
  Max Deflection/1 -> Out1/1  "dV"
  D-Pitch/1 -> I-Pitch5/1
  Target Pitch/1 -> Add9/1
  Add10/1 -> Rate Limiter Dynamic/2
  Rate Limiter Dynamic/1 -> Max Deflection/1
  Constant/1 -> Rate Limiter Dynamic/1
  Constant1/1 -> Rate Limiter Dynamic/3
  Target Depth/1 -> Add7/1
  I-Pitch/1 -> I-Pitch1/1
  I-Depth/1 -> I-Pitch2/1
  Mux/1 -> Out2/1
  I-Pitch1/1 -> Add1/2
  I-Pitch2/1 -> Add/2
  I-Pitch3/1 -> Add1/1
  I-Pitch4/1 -> Add/1
  I-Pitch5/1 -> Add1/3
  I-Pitch6/1 -> Add/3

== system Model_6DOF_B3/Controller/n:RPS PID ==
  ref. Velocity : Inport
  Current Velocity : Inport  Port=2
  Add : Sum  Inputs=+++
  Add1 : Sum  Inputs=-+
  Constant1 : Constant  Value=4
  Divide : Product  Inputs=*/
  Gain1 : Gain  Gain=14.65
  Gain4 : Gain  Gain=1.465
  Integrator : Integrator
  Rate Limiter Dynamic : simulink/Discontinuities/Rate Limiter Dynamic
  Rate Max : Constant  Value=14.65
  Rate Min : Constant  Value=-14.65
  Saturation6 : Saturate  UpperLimit=10  LowerLimit=0.01
  Selector : Selector  InputPortWidth=6  IndexOptions=Index vector (dialog)  Indices=1  OutputSizes=1
  Out1 : Outport  VectorParamsAs1DForOutWhenUnconnected=off
  wires:
  Selector/1 -> Add1/2  "current"
  Constant1/1 -> Divide/2
  ref. Velocity/1 -> Add1/1, Divide/1  "target"
  Add1/1 -> Gain1/1, Integrator/1  "error term"
  Current Velocity/1 -> Selector/1
  Gain4/1 -> Add/3
  Gain1/1 -> Add/2
  Add/1 -> Rate Limiter Dynamic/2
  Divide/1 -> Add/1
  Rate Limiter Dynamic/1 -> Saturation6/1
  Rate Max/1 -> Rate Limiter Dynamic/1
  Rate Min/1 -> Rate Limiter Dynamic/3
  Integrator/1 -> Gain4/1
  Saturation6/1 -> Out1/1

== system Model_6DOF_B3/HDM 6DOF V1/Effective Veloicity Calclation ==
  Bv : Inport
  uwsXi : Inport  Port=2
  uwsCG : Inport  Port=3
  Add{,1..4} (5 alike) : Sum
  Demux : Demux  Outputs=5
  Demux1 : Demux  Outputs=3
  Demux2 : Demux  Outputs=5
  Gain : Gain  Gain=0
  Gain1 : Gain  Gain=0
  Gain2 : Gain  Gain=0
  MATLAB Function : MATLAB Function  TreatAsAtomicUnit=on
  MATLAB Function1 : MATLAB Function  TreatAsAtomicUnit=on
  MATLAB Function2 : MATLAB Function  TreatAsAtomicUnit=on
  X_SP1 : Constant  Value=[31.924; 3.861; -3.861;]
  X_SP2 : Constant  Value=[31.924; 3.861; 3.861;]
  X_SP3 : Constant  Value=[31.924; -3.861; 3.861;]
  X_SP4 : Constant  Value=[31.924; -3.861; -3.861;]
  X_XB : Constant  Value=[-10.465; 0; 9.732;]
  aX : Scope  NumInputPorts=5
  n1 : Constant  Value=[0; 1/sqrt(2); -1/sqrt(2);]
  n2 : Constant  Value=[0; 1/sqrt(2); 1/sqrt(2);]
  n3 : Constant  Value=[0; -1/sqrt(2); 1/sqrt(2);]
  n4 : Constant  Value=[0; -1/sqrt(2); -1/sqrt(2);]
  n5 : Constant  Value=[0; 1; 0;]
  nh : Constant  Value=[-1; 0; 0;]
  urXi : Scope  NumInputPorts=5
  Alpha : Outport
  Beta : Outport  Port=2
  Umag : Outport  Port=3
  aXi : Outport  Port=4
  UeX : Outport  Port=5
  wires:
  Bv/1 -> MATLAB Function1/6(U_ship), MATLAB Function2/1(Bv)
  nh/1 -> MATLAB Function/1(nh)
  n1/1 -> MATLAB Function/2(n1)
  n2/1 -> MATLAB Function/3(n2)
  n3/1 -> MATLAB Function/4(n3)
  n4/1 -> MATLAB Function/5(n4)
  X_XB/1 -> MATLAB Function1/5(rXB)
  X_SP2/1 -> MATLAB Function1/2(rX2)
  X_SP3/1 -> MATLAB Function1/3(rX3)
  X_SP4/1 -> MATLAB Function1/4(rX4)
  X_SP1/1 -> MATLAB Function1/1(rX1)
  n5/1 -> MATLAB Function/6(nB)
  MATLAB Function1/1(urX1) -> Add/1, urXi/1
  MATLAB Function/1(aX) -> Gain1/1, Demux2/1
  Demux/1 -> Add/2
  Add/1 -> MATLAB Function/7(urX1)
  Add1/1 -> MATLAB Function/8(urX2)
  Add2/1 -> MATLAB Function/9(urX3)
  Add3/1 -> MATLAB Function/10(urX4)
  Add4/1 -> MATLAB Function/11(urXB)
  Demux/2 -> Add1/2
  Demux/3 -> Add2/2
  Demux/4 -> Add3/2
  Demux/5 -> Add4/2
  MATLAB Function1/5(urXB) -> Add4/1, urXi/5
  MATLAB Function1/4(urX4) -> Add3/1, urXi/4
  MATLAB Function1/3(urX3) -> Add2/1, urXi/3
  MATLAB Function1/2(urX2) -> Add1/1, urXi/2
  MATLAB Function2/1(alpha) -> Gain/1
  MATLAB Function2/2(beta) -> Beta/1
  MATLAB Function2/3(Umag) -> Umag/1
  MATLAB Function/2(UeX) -> UeX/1
  Demux1/1 -> MATLAB Function2/2(uCG)
  Demux1/2 -> MATLAB Function2/3(vCG)
  Demux1/3 -> MATLAB Function2/4(wCG)
  Demux2/1 -> aX/1
  Demux2/2 -> aX/2
  Demux2/3 -> aX/3
  Demux2/4 -> aX/4
  Demux2/5 -> aX/5
  uwsCG/1 -> Demux1/1
  Gain/1 -> Alpha/1
  Gain1/1 -> aXi/1
  Gain2/1 -> Demux/1
  uwsXi/1 -> Gain2/1

== system Model_6DOF_B3/HDM 6DOF V1/Effective dX Calculation ==
  dX CTRL : Inport
  aXi : Inport  Port=2
  Add{,1..4} (5 alike) : Sum
  Demux : Demux  Outputs=5
  Demux1 : Demux  Outputs=5
  Mux6 : Mux  Inputs=5
  dXeff : Outport
  wires:
  dX CTRL/1 -> Demux/1
  aXi/1 -> Demux1/1
  Add/1 -> Mux6/1
  Add1/1 -> Mux6/2
  Add2/1 -> Mux6/3
  Add3/1 -> Mux6/4
  Add4/1 -> Mux6/5
  Demux/1 -> Add/1
  Demux/2 -> Add1/1
  Demux/3 -> Add2/1
  Demux/4 -> Add3/1
  Demux/5 -> Add4/1
  Demux1/1 -> Add/2
  Demux1/2 -> Add1/2
  Demux1/3 -> Add2/2
  Demux1/4 -> Add3/2
  Demux1/5 -> Add4/2
  Mux6/1 -> dXeff/1

== system Model_6DOF_B3/HDM 6DOF V1/K ==
  Bx : Inport
  Bv : Inport  Port=2
  Ba : Inport  Port=3
  Beta : Inport  Port=4
  Umag : Inport  Port=5
  dX : Inport  Port=6
  UeX : Inport  Port=7
  dLCG : Inport  Port=8
  dmass : Inport  Port=9
  Kvm : Inport  Port=10
  Abs : Abs
  Abs1 : Abs
  Abs2 : Abs
  K'p|p| : Lookup_n-D  NumberOfTableDimensions=1  BreakpointsForDimension1=|  Table=|  InternalRulePriority=Speed  RndMeth=Simplest  InputSameDT=on
      BreakpointsForDimension1=|
      | [-0.0015
      | -0.0012
      | -0.0009
      | -0.0006
      | -0.0003
      | -0.0001
      | 0.0001
      | 0.0003
      | 0.0006
      | 0.0009
      | 0.0012
      | 0.0015]
      Table=|
      | [-1.3011E-02
      | -1.6962E-02
      | -2.0682E-02
      | -3.1419E-02
      | -6.4407E-02
      | -1.9322E-01
      | 1.9322E-01
      | 6.4378E-02
      | 3.1944E-02
      | 2.1072E-02
      | 1.6415E-02
      | 1.3407E-02]
  K'up : Lookup_n-D  NumberOfTableDimensions=1  BreakpointsForDimension1=|  Table=|  InternalRulePriority=Speed  RndMeth=Simplest  InputSameDT=on
      BreakpointsForDimension1=|
      | [0.03999989
      | 0.079999993
      | 0.11999963
      | 0.15999956]
      Table=|
      | [-4.0344E-04
      | -8.1402E-04
      | -1.2116E-03
      | -1.6125E-03]
  K'ur : Lookup_n-D  NumberOfTableDimensions=1  BreakpointsForDimension1=|  Table=|  InternalRulePriority=Speed  RndMeth=Simplest  InputSameDT=on
      BreakpointsForDimension1=|
      | [-0.0015
      | -0.0012
      | -0.0009
      | -0.0006
      | -0.0003
      | -0.0001
      | 0.0001
      | 0.0003
      | 0.0006
      | 0.0009
      | 0.0012
      | 0.0015]
      Table=|
      | [-1.3011E-02
      | -1.6962E-02
      | -2.0682E-02
      | -3.1419E-02
      | -6.4407E-02
      | -1.9322E-01
      | 1.9322E-01
      | 6.4378E-02
      | 3.1944E-02
      | 2.1072E-02
      | 1.6415E-02
      | 1.3407E-02]
  K'uvw : Lookup_n-D  NumberOfTableDimensions=3  BreakpointsForDimension1=|  BreakpointsForDimension2=|  BreakpointsForDimension3=|  Table=|  InternalRulePriority=Speed  RndMeth=Simplest  InputSameDT=on
      BreakpointsForDimension1=|
      | [0
      | 4
      | 8
      | 12]
      BreakpointsForDimension2=|
      | [-5.1444E+00
      | -3.0866E+00
      | -1.5433E+00
      | ]
      Table=|
      | reshape([0.0000000E+00
      | 1.5570290E-04
      | 3.7677829E-04
      | 6.0025374E-04
      | 0.0000000E+00
      | 1.5575678E-04
      | 3.8557685E-04
      | 6.0103850E-04
      | 0.0000000E+00
      | 1.7511088E-04
      | 3.8376789E-04
      | 6.0108480E-04
      | 0.0000000E+00
      | 1.9071552E-04
      | 4.0986649E-04
      | 6.4012030E-04
      | 0.0000000E+00
      | 1.8940622E-04
      | 4.0946931E-04
      | 6.3613461E-04
      | 0.0000000E+00
      | 1.8621071E-04
      | 4.0619654E-04
      | 7.0286379E-04
      | 0.0000000E+00
      | 2.0712189E-04
      | 4.4751988E-04
      | 7.0514631E-04
      | 0.0000000E+00
      | 1.9895751E-04
      | 4.3099356E-04
      | 6.6994571E-04
      | 0.0000000E+00
      | 1.9568554E-04
      | 4.2679977E-04
      | 6.6445067E-04
      | 0.0000000E+00
      | 2.4359563E-04
      | 5.3740096E-04
      | 8.5879902E-04
      | 0.0000000E+00
      | 2.0890025E-04
      | 4.5502130E-04
      | 7.1388224E-04
      | 0.0000000E+00
      | 2.0575072E-04
      | 4.5505766E-04
      | 7.0285206E-04],[4,3,4])
      BreakpointsForDimension3=|
      | [-35.0624 -18.3724 -15.3724 -13.8724
      | ]
      settings: InputPortMap=u0,u1,u2
  KdXi : Subsystem
  Mux : Mux
  Mx : MATLAB Function  TreatAsAtomicUnit=on
  Product{,1..2,4..5} (5 alike) : Product
  Scope : Scope
  Scope1 : Scope
  Selector10 : Selector  InputPortWidth=6  IndexOptions=Index vector (dialog)  Indices=1  OutputSizes=1
  Selector2 : Selector  InputPortWidth=6  IndexOptions=Index vector (dialog)  Indices=3  OutputSizes=1
  Selector4 : Selector  InputPortWidth=6  IndexOptions=Index vector (dialog)  Indices=4  OutputSizes=1
  Selector8 : Selector  InputPortWidth=6  IndexOptions=Index vector (dialog)  Indices=2  OutputSizes=1
  Sign : Signum
  Sign1 : Signum
  To Workspace : ToWorkspace  VariableName=K_total  SaveFormat=Timeseries  SampleTime=-1
  To Workspace1 : ToWorkspace  VariableName=K_hull  SaveFormat=Timeseries  SampleTime=-1
  To Workspace2 : ToWorkspace  VariableName=KdX  SaveFormat=Timeseries  SampleTime=-1
  To Workspace3 : ToWorkspace  VariableName=KApp  SaveFormat=Timeseries  SampleTime=-1
  K : Outport
  wires:
  Bv/1 -> Selector10/1, Selector4/1, Selector8/1, Mx/2(Bv)
  Bx/1 -> Mx/1(Bx), Selector2/1
  Selector10/1 -> K'uvw/2, Product1/1
  Ba/1 -> Mx/3(Ba)
  UeX/1 -> Mx/9(UeX)
  Beta/1 -> Sign1/1, Abs2/1
  Umag/1 -> Mx/8(Umag)
  dLCG/1 -> Mx/10(dLCG)
  dmass/1 -> Mx/11(dmass)
  dX/1 -> KdXi/1(dX)
  K'up/1 -> Product/2
  K'p|p|/1 -> Mx/5(CKur)
  Product4/1 -> K'ur/1
  Selector8/1 -> Product4/1
  Abs/1 -> Product5/1
  Product5/1 -> K'p|p|/1
  Selector4/1 -> Product1/2, Product5/2, Abs/1, Product4/2
  K'ur/1 -> Mx/6(CKpp)
  Mx/1(K) -> Scope/1, To Workspace/1, K/1
  KdXi/1(KdXi) -> Mx/12(CNdXi)
  Selector2/1 -> KdXi/2(z), K'uvw/3
  K'uvw/1 -> Product2/2
  Product1/1 -> Sign/1, Abs1/1
  Abs1/1 -> K'up/1
  Sign/1 -> Product/1
  Product/1 -> Mx/4(CKup)
  Product2/1 -> Scope1/1, Mx/7(CKuvw)
  Abs2/1 -> K'uvw/1
  Sign1/1 -> Product2/1
  Mx/6(K_hull) -> To Workspace1/1
  Mux/1 -> To Workspace2/1
  Mx/2(KdX1) -> Mux/1
  Mx/3(KdX2) -> Mux/2
  Mx/4(KdX3) -> Mux/3
  Mx/5(KdX4) -> Mux/4
  Mx/7(KApp) -> To Workspace3/1
  Kvm/1 -> Mx/13(Kvm)

== system Model_6DOF_B3/HDM 6DOF V1/M ==
  Bx : Inport
  Bv : Inport  Port=2
  Ba : Inport  Port=3
  Alpha : Inport  Port=4
  Umag : Inport  Port=5
  dX : Inport  Port=6
  UeSP : Inport  Port=7
  dLCG : Inport  Port=8
  dmass : Inport  Port=9
  Mvm : Inport  Port=10
  Add : Sum
  Constant : Constant  Value=0
  Constant1 : Constant  Value=2.4400E-05
  Gain : Gain  Gain=0.5
  M'prop : Lookup_n-D  NumberOfTableDimensions=1  BreakpointsForDimension1=[-7.7166666 -5.1444444 -3.08666664]  Table=[-0.00022 -0.0002 -0.00015]  InternalRulePriority=Speed  RndMeth=Simplest  InputSameDT=on
  M'uvw1 : Lookup_n-D  NumberOfTableDimensions=3  BreakpointsForDimension1=|  BreakpointsForDimension2=|  BreakpointsForDimension3=|  Table=|  InternalRulePriority=Speed  RndMeth=Simplest  InputSameDT=on
      BreakpointsForDimension1=|
      | [-12
      | -8
      | -4
      | 0
      | 4
      | 8
      | 12]
      BreakpointsForDimension2=|
      | [-5.1444E+00
      | -3.0866E+00
      | -1.5433E+00
      | ]
      Table=|
      | reshape([-2.40251E-03
      | -1.59538E-03
      | -8.21748E-04
      | -3.60182E-06
      | 8.13350E-04
      | 1.50586E-03
      | 2.39707E-03
      | -2.43392E-03
      | -1.61509E-03
      | -8.50748E-04
      | -3.60182E-06
      | 8.24271E-04
      | 1.51842E-03
      | 2.43805E-03
      | -2.45014E-03
      | -1.65711E-03
      | -9.11210E-04
      | -3.60182E-06
      | 8.61300E-04
      | 1.57459E-03
      | 2.42777E-03
      | -2.54380E-03
      | -1.68842E-03
      | -8.33041E-04
      | 2.23377E-05
      | 8.77717E-04
      | 1.73310E-03
      | 2.58847E-03
      | -2.63734E-03
      | -1.75078E-03
      | -8.64221E-04
      | 2.23377E-05
      | 9.08896E-04
      | 1.79546E-03
      | 2.68201E-03
      | -2.83738E-03
      | -1.88414E-03
      | -9.30902E-04
      | 2.23377E-05
      | 9.75577E-04
      | 1.92882E-03
      | 2.88206E-03
      | -2.63786E-03
      | -1.74504E-03
      | -8.52211E-04
      | 4.06140E-05
      | 9.33439E-04
      | 1.82626E-03
      | 2.71909E-03
      | -2.63728E-03
      | -1.74465E-03
      | -8.52017E-04
      | 4.06140E-05
      | 9.33245E-04
      | 1.82588E-03
      | 2.71851E-03
      | -2.86138E-03
      | -1.89405E-03
      | -9.26716E-04
      | 4.06140E-05
      | 1.00794E-03
      | 1.97527E-03
      | 2.94260E-03
      | -0.002723494
      | -0.001792522
      | -0.000861549
      | 6.9423E-05
      | 0.001000396
      | 0.001931368
      | 0.002862341
      | -0.002736476
      | -0.001798489
      | -0.000860502
      | 6.9423E-05
      | 0.001015473
      | 0.00195346
      | 0.002891447
      | -0.002765582
      | -0.00182058
      | -0.000875579
      | 6.9423E-05
      | 0.001014425
      | 0.001959426
      | 0.002904428],[7,3,4])
      BreakpointsForDimension3=|
      | [-35.0624 -18.3724 -15.3724 -13.8724
      | ]
      settings: InputPortMap=u0,u1,u2
  MATLAB Function2 : MATLAB Function  TreatAsAtomicUnit=on
  Mdxi : Subsystem
  Mqq2 : Lookup_n-D  NumberOfTableDimensions=1  BreakpointsForDimension1=|  Table=|  InternalRulePriority=Speed  RndMeth=Simplest  InputSameDT=on
      BreakpointsForDimension1=|
      | [-0.02
      | -0.015
      | -0.012958963
      | -0.009719222
      | -0.006479482
      | -0.003239741
      | -0.00161987
      | -0.000647948
      | 0.000647948
      | 0.00161987
      | 0.003239741
      | 0.006479482
      | 0.009719222
      | 0.012958963
      | 0.015
      | 0.02
      | ]
      Table=|
      | [-2.2571E-03
      | -2.3029E-03
      | -2.0965E-03
      | -2.0229E-03
      | -2.1546E-03
      | -1.4789E-03
      | -1.5664E-03
      | -1.4544E-03
      | -1.4705E-03
      | -1.4942E-03
      | -1.8790E-03
      | -1.8821E-03
      | -2.1009E-03
      | -2.0521E-03
      | -2.1685E-03
      | -2.0822E-03
      | ]
  Muq : Lookup_n-D  BreakpointsForDimension1=|  BreakpointsForDimension2=|  Table=|  InternalRulePriority=Speed  RndMeth=Simplest  InputSameDT=on
      BreakpointsForDimension1=|
      | [-2.00E-01
      | -1.50E-01
      | -1.00E-01
      | -5.00E-02
      | 0.00E+00
      | 5.00E-02
      | 1.00E-01
      | 1.50E-01
      | 2.00E-01
      | ]
      Table=|
      | reshape([-3.95902E-04
      | -2.96922E-04
      | -1.97952E-04
      | -9.89720E-05
      | 0.00000E+00
      | 9.89750E-05
      | 1.97948E-04
      | 2.96928E-04
      | 3.95898E-04
      | -4.94864E-04
      | -3.71144E-04
      | -2.47434E-04
      | -1.23714E-04
      | 0.00000E+00
      | 1.23715E-04
      | 2.47426E-04
      | 3.71146E-04
      | 4.94856E-04
      | -5.69298E-04
      | -4.26978E-04
      | -2.84648E-04
      | -1.42328E-04
      | 0.00000E+00
      | 1.42322E-04
      | 2.84652E-04
      | 4.26972E-04
      | 5.69302E-04
      | -5.60922E-04
      | -4.20692E-04
      | -2.80462E-04
      | -1.40232E-04
      | 0.00000E+00
      | 1.40228E-04
      | 2.80458E-04
      | 4.20688E-04
      | 5.60918E-04],[9,4])
      BreakpointsForDimension2=|
      | [-7.7166 -5.1444 -3.08664 -1.54332
      | ]
      settings: InputPortMap=u0,u1
  Mux : Mux  Inputs=6
  Mwq : Lookup_n-D  NumberOfTableDimensions=1  BreakpointsForDimension1=|  Table=|  InternalRulePriority=Speed  RndMeth=Simplest  InputSameDT=on
      BreakpointsForDimension1=|
      | [-0.0015
      | -0.0012
      | -0.0009
      | -0.0006
      | -0.0003
      | -0.0001
      | 0.0001
      | 0.0003
      | 0.0006
      | 0.0009
      | 0.0012
      | 0.0015]
      Table=|
      | [-1.3011E-02
      | -1.6962E-02
      | -2.0682E-02
      | -3.1419E-02
      | -6.4407E-02
      | -1.9322E-01
      | 1.9322E-01
      | 6.4378E-02
      | 3.1944E-02
      | 2.1072E-02
      | 1.6415E-02
      | 1.3407E-02]
  My : MATLAB Function  TreatAsAtomicUnit=on
  Product4 : Product
  Product5 : Product
  Saturation2 : Saturate  UpperLimit=0.0015  LowerLimit=-0.0015
  Saturation3 : Saturate  UpperLimit=0.02  LowerLimit=-0.02
  Saturation4 : Saturate  UpperLimit=-13.8724  LowerLimit=-35.0624
  Scope1 : Scope
  Scope2 : Scope
  Selector10 : Selector  InputPortWidth=6  IndexOptions=Index vector (dialog)  Indices=1  OutputSizes=1
  Selector2 : Selector  InputPortWidth=6  IndexOptions=Index vector (dialog)  Indices=3  OutputSizes=1
  Selector4 : Selector  InputPortWidth=6  IndexOptions=Index vector (dialog)  Indices=5  OutputSizes=1
  Selector8 : Selector  InputPortWidth=6  IndexOptions=Index vector (dialog)  Indices=3  OutputSizes=1
  To Workspace8 : ToWorkspace  VariableName=Benchmark_M  SaveFormat=Timeseries  SampleTime=-1
  M : Outport
  wires:
  M'uvw1/1 -> Gain/1
  Selector2/1 -> Saturation4/1
  Mvm/1 -> Mux/5, My/14(Mvm)
  Mdxi/1(MdX) -> Scope1/1, My/13(MdXi)
  My/1(MY) -> Mux/6, M/1
  Muq/1 -> My/6(Muq)
  Saturation3/1 -> Mqq2/1
  Saturation2/1 -> Mwq/1
  MATLAB Function2/1(y) -> Product5/1
  Selector8/1 -> Product5/2
  Product5/1 -> Saturation2/1
  Product4/1 -> Muq/1
  Mwq/1 -> My/5(Mwq)
  Mqq2/1 -> My/4(Mqq)
  dX/1 -> Scope2/1, Mdxi/1(dX)
  dmass/1 -> My/12(dmass)
  dLCG/1 -> My/11(dLCG)
  Umag/1 -> My/9(Umag)
  Alpha/1 -> M'uvw1/1
  Selector4/1 -> Product4/2, Saturation3/1, MATLAB Function2/1(u)
  UeSP/1 -> My/10(UeSP)
  M'prop/1 -> My/7("Mprop ")
  Ba/1 -> My/3(Ba)
  Selector10/1 -> M'uvw1/2, M'prop/1, Product4/1, Muq/2
  Bx/1 -> Selector2/1, My/1(Bx)
  Bv/1 -> My/2(Bv), Selector8/1, Selector4/1, Selector10/1
  Constant/1 -> My/15(M_ext)
  My/2(MYApp) -> Mux/1
  My/3(MYStat) -> ?
  My/4(Mprop) -> Mux/4
  My/5(M_hull) -> Mux/2
  My/6(MYuvw) -> ?
  Saturation4/1 -> Mdxi/2(z), M'uvw1/3
  My/7(MY_hyd) -> Mux/3
  Gain/1 -> Add/1
  Add/1 -> My/8(Muvw)
  Constant1/1 -> Add/2
  Mux/1 -> To Workspace8/1
